simulink model "FID_Generator"  (R2020b)
settings: Solver=VariableStepAuto  StartTime=0.0  StopTime=.00015  RelTol=1e-3
libraries: fl_lib x2, nesl_utility x1
settings Model: Creator=jaket  LastModifiedBy=jaket

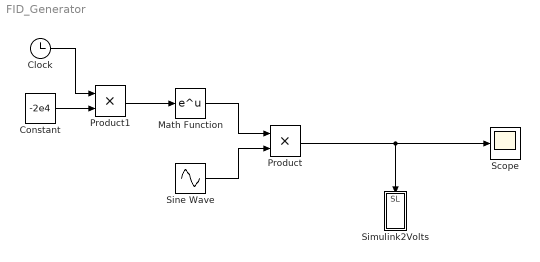
== system FID_Generator ==
  Clock : Clock
  Constant : Constant  Value=-2e4
  Math Function : Math  SaturateOnIntegerOverflow=on
  Product : Product
  Product1 : Product
  Scope : Scope
  Simulink2Volts : Subsystem
  Sine Wave : Sin  Amplitude=10e-6  Frequency=135383793  SampleTime=0
  wires:
  Clock/1 -> Product1/1
  Constant/1 -> Product1/2
  Product1/1 -> Math Function/1
  Math Function/1 -> Product/1
  Sine Wave/1 -> Product/2
  Product/1 -> Simulink2Volts/1(SL), Scope/1

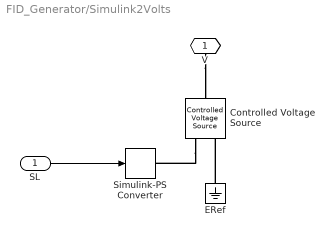
== system FID_Generator/Simulink2Volts ==
  SL : Inport
  Controlled Voltage Source : fl_lib/Electrical/Electrical Sources/Controlled Voltage Source
      settings: SourceProductName=Foundation Library
  ERef : fl_lib/Electrical/Electrical Elements/Electrical Reference
      settings: SourceProductName=Foundation Library
  Simulink-PS Converter : nesl_utility/Simulink-PS Converter  PhysicalDomain=network_engine_domain  SubClassName=ps_input  LeftPortType=input  RightPortType=output  PseudoPeriodic=off  Frequencies=[]  NoiseDistribution=none  NoiseParameters=[]  Unit=V  AffineConversion=off  FilteringAndDerivatives=zero  SimscapeFilterOrder=1  InputFilterTimeConstant=.001  UdotUserProvided=0
      settings: SourceProductName=Utilities
  V : PMIOPort  Side=Right
  wires:
  SL/1 -> Simulink-PS Converter/1
  connections:
  V/RConn1 -- Controlled Voltage Source/LConn1
  ERef/LConn1 -- Controlled Voltage Source/RConn2
  Controlled Voltage Source/RConn1 -- Simulink-PS Converter/RConn1
